simulink model "RLC"  (R2015b)
settings: Solver=VariableStepAuto  StartTime=0.0  StopTime=1  RelTol=1e-3
values from neighbouring files (symbols this model uses):
  C = [1 0 0 0]    [Parametri.m]
  R = 1    [Parametri.m]
undefined symbols (not defined in the file or in its folder): L
settings Model: Creator=user  LastModifiedBy=user

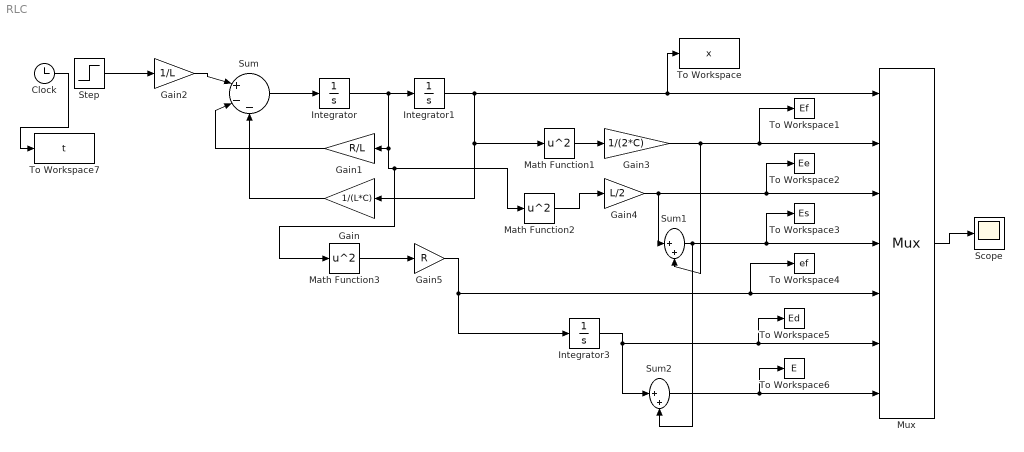
== system RLC ==
  Clock : Clock
  Gain : Gain  Gain=1/(L*C)
  Gain1 : Gain  Gain=R/L
  Gain2 : Gain  Gain=1/L
  Gain3 : Gain  Gain=1/(2*C)
  Gain4 : Gain  Gain=L/2
  Gain5 : Gain  Gain=R
  Integrator : Integrator
  Integrator1 : Integrator
  Integrator3 : Integrator
  Math Function1 : Math  Operator=square  SaturateOnIntegerOverflow=on
  Math Function2 : Math  Operator=square  SaturateOnIntegerOverflow=on
  Math Function3 : Math  Operator=square  SaturateOnIntegerOverflow=on
  Mux : Mux  Inputs=7
  Scope : Scope
  Step : Step  Before=0.5  After=0  SampleTime=0
  Sum : Sum  Inputs=|+--
  Sum1 : Sum  Inputs=|++
  Sum2 : Sum  Inputs=|++
  To Workspace : ToWorkspace  VariableName=x  SampleTime=-1
  To Workspace1 : ToWorkspace  VariableName=Ef  SampleTime=-1
  To Workspace2 : ToWorkspace  VariableName=Ee  SampleTime=-1
  To Workspace3 : ToWorkspace  VariableName=Es  SampleTime=-1
  To Workspace4 : ToWorkspace  VariableName=ef  SampleTime=-1
  To Workspace5 : ToWorkspace  VariableName=Ed  SampleTime=-1
  To Workspace6 : ToWorkspace  VariableName=E  SampleTime=-1
  To Workspace7 : ToWorkspace  VariableName=t  SampleTime=-1
  wires:
  Sum/1 -> Integrator/1
  Integrator1/1 -> Math Function1/1, Gain/1, Mux/1, To Workspace/1
  Gain/1 -> Sum/3
  Gain1/1 -> Sum/2
  Step/1 -> Gain2/1
  Gain2/1 -> Sum/1
  Clock/1 -> To Workspace7/1
  Math Function1/1 -> Gain3/1
  Gain3/1 -> Sum1/2, Mux/2, To Workspace1/1
  Integrator/1 -> Math Function3/1, Math Function2/1, Gain1/1, Integrator1/1
  Math Function2/1 -> Gain4/1
  Gain4/1 -> Sum1/1, Mux/3, To Workspace2/1
  Sum1/1 -> Mux/4, To Workspace3/1, Sum2/2
  Integrator3/1 -> Sum2/1, Mux/6, To Workspace5/1
  Sum2/1 -> Mux/7, To Workspace6/1
  Mux/1 -> Scope/1
  Gain5/1 -> Integrator3/1, Mux/5, To Workspace4/1
  Math Function3/1 -> Gain5/1
